simulink model "Example_VR_Simulation"  (Simulink 8.0)
settings: Solver=ode45  StartTime=0.0  StopTime=35  RelTol=1e-3
libraries: vrlib x6
settings Model: Creator=ajn5049  LastModifiedBy=ajn5049

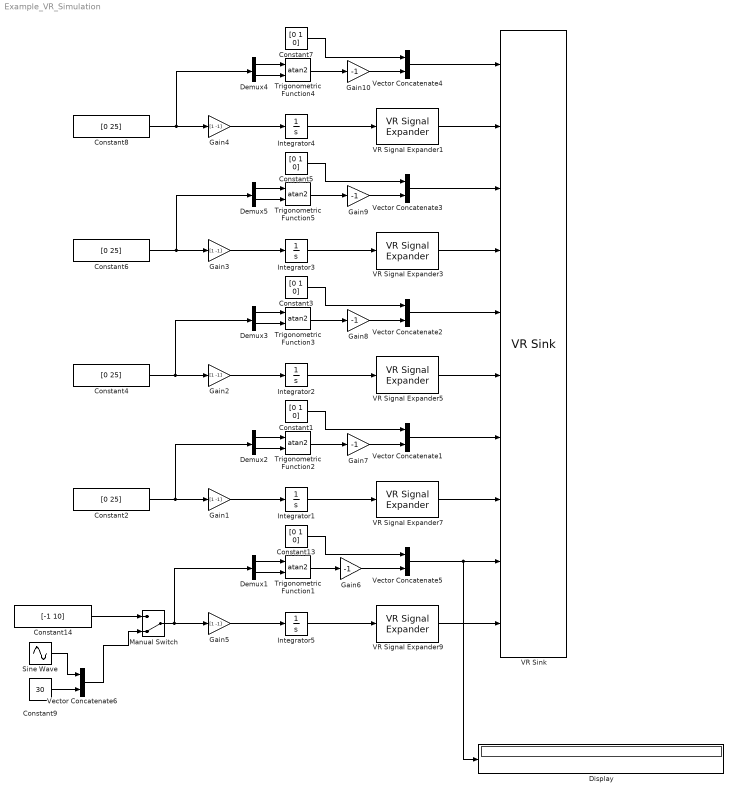
== system Example_VR_Simulation ==
  Constant{1,3,5,7,13} (5 alike) : Constant  Value=[0 1 0]
  Constant14 : Constant  Value=[-1 10]
  Constant{2,4,6,8} (4 alike) : Constant  Value=[0 25]
  Constant9 : Constant  Value=30
  Demux{1..5} (5 alike) : Demux  Outputs=2
  Display : Display
  Gain{1..5} (5 alike) : Gain  Gain=[1 -1]
  Gain{6..10} (5 alike) : Gain  Gain=-1
  Integrator{1..4} (4 alike) : Integrator  InitialCondition=[0, 0]
  Integrator5 : Integrator  InitialCondition=[-3.66/2, 0]
  Manual Switch : ManualSwitch  CurrentSetting=0
  Sine Wave : Sin  Amplitude=2  Phase=pi/2  SampleTime=0
  Trigonometric Function{1..5} (5 alike) : Trigonometry  Operator=atan2
  VR Signal Expander{1,3,5,7,9} (5 alike) : vrlib/VR Signal Expander  outwidth=3  outidx=[1 3]
  VR Sink : vrlib/VR Sink  InstantiateOnLoad=on  SampleTime=0.1  ViewEnable=on  RemoteChange=off  RemoteView=off  FieldsWritten=Lotus.rotation.4.1.1.double#Lotus.translation.3.1.1.double#Alfa_Romeo.rotation.4.1.1.double#Alfa_Romeo.translation.3.1.1.double#Logging_Truck.rotation.4.1.1.double#Logging_Truck.translation.3.1.1.double#Mustang.rotation.4.1.1.double#Mustang.translation.3.1.1.double#Octavia.rotation.4.1.1.double#Octavia.translation.3.1.1.double  WorldFileName=C:\Other\Virtual Worlds\VR_Simulation.wrl  WorldDescription=Simple Highway Model  AutoView=on  VideoDimensions=[200 320]*2  AllowVariableSize=off  FigureProperties="{'Position', 'Name', 'Viewpoint', 'CameraBound', 'CameraDirection', 'CameraPosition', 'CameraUpVector', 'ZoomFactor', 'Antialiasing', 'Headlight', 'Lighting', 'NavPanel', 'StatusBar', 'ToolBar', 'Textures', 'Transparency', 'Triad', 'Wireframe', 'NavZones', 'NavMode', 'NavSpeed', 'CaptureFileFormat', 'CaptureFileName', 'Record2DCompressMethod', 'Record2DCompressQuality', 'Record2D', 'Record2DFileName', 'Record2DFPS'; [5.0000000000000000e+00   9.2000000000000000e+01   5.7600000000000000e+02   3.8000000000000000e+02], 'Simple Highway Model', 'Car1 - View from Behind - Rot', 'on', [0.0000000000000000e+00   0.0000000000000000e+00  -1.0000000000000000e+00], [0.0000000000000000e+00   0.0000000000000000e+00   0.0000000000000000e+00], [0.0000000000000000e+00   1.0000000000000000e+00   0.0000000000000000e+00], [1.0000000000000000e+00], 'on', 'on', 'on', 'halfbar', 'on', 'on', 'on', 'on', 'none', 'off', 'off', 'walk', 'normal', 'tif', '%f_anim_%n.tif', 'auto', [7.5000000000000000e+01], 'off', '%f_anim_%n.avi', [1.5000000000000000e+01]; [5.8600000000000000e+02   6.0000000000000000e+01   6.4000000000000000e+02   4.0000000000000000e+02], 'Simple Highway Model', 'Car1 - View from Above Ahead - Rot', 'on', [0.0000000000000000e+00   0.0000000000000000e+00  -1.0000000000000000e+00], [0.0000000000000000e+00   0.0000000000000000e+00   0.0000000000000000e+00], [0.0000000000000000e+00   1.0000000000000000e+00   0.0000000000000000e+00], [1.0000000000000000e+00], 'on', 'on', 'on', 'none', 'off', 'off', 'on', 'on', 'none', 'off', 'off', 'walk', 'normal', 'tif', '%f_anim_%n.tif', 'auto', [7.5000000000000000e+01], 'off', '***video***', [1.5000000000000000e+01]}"
  Vector Concatenate{1..6} (6 alike) : Concatenate
  wires:
  Trigonometric Function1/1 -> Gain6/1
  Constant13/1 -> Vector Concatenate5/1
  Integrator5/1 -> VR Signal Expander9/1
  Gain5/1 -> Integrator5/1
  Vector Concatenate4/1 -> VR Sink/1
  Vector Concatenate1/1 -> VR Sink/7
  VR Signal Expander5/1 -> VR Sink/6
  VR Signal Expander7/1 -> VR Sink/8
  Vector Concatenate5/1 -> Display/1, VR Sink/9
  Vector Concatenate2/1 -> VR Sink/5
  VR Signal Expander3/1 -> VR Sink/4
  VR Signal Expander9/1 -> VR Sink/10
  Vector Concatenate3/1 -> VR Sink/3
  VR Signal Expander1/1 -> VR Sink/2
  Trigonometric Function2/1 -> Gain7/1
  Constant1/1 -> Vector Concatenate1/1
  Integrator1/1 -> VR Signal Expander7/1
  Gain1/1 -> Integrator1/1
  Trigonometric Function3/1 -> Gain8/1
  Constant3/1 -> Vector Concatenate2/1
  Integrator2/1 -> VR Signal Expander5/1
  Gain2/1 -> Integrator2/1
  Constant6/1 -> Demux5/1, Gain3/1
  Integrator3/1 -> VR Signal Expander3/1
  Gain3/1 -> Integrator3/1
  Trigonometric Function4/1 -> Gain10/1
  Constant7/1 -> Vector Concatenate4/1
  Constant8/1 -> Demux4/1, Gain4/1
  Integrator4/1 -> VR Signal Expander1/1
  Gain4/1 -> Integrator4/1
  Demux4/1 -> Trigonometric Function4/1
  Demux4/2 -> Trigonometric Function4/2
  Vector Concatenate6/1 -> Manual Switch/2
  Demux1/1 -> Trigonometric Function1/1
  Demux1/2 -> Trigonometric Function1/2
  Constant2/1 -> Demux2/1, Gain1/1
  Demux2/1 -> Trigonometric Function2/1
  Demux2/2 -> Trigonometric Function2/2
  Constant4/1 -> Demux3/1, Gain2/1
  Demux3/1 -> Trigonometric Function3/1
  Demux3/2 -> Trigonometric Function3/2
  Trigonometric Function5/1 -> Gain9/1
  Demux5/1 -> Trigonometric Function5/1
  Demux5/2 -> Trigonometric Function5/2
  Constant5/1 -> Vector Concatenate3/1
  Gain6/1 -> Vector Concatenate5/2
  Gain7/1 -> Vector Concatenate1/2
  Gain8/1 -> Vector Concatenate2/2
  Gain9/1 -> Vector Concatenate3/2
  Gain10/1 -> Vector Concatenate4/2
  Manual Switch/1 -> Demux1/1, Gain5/1
  Constant14/1 -> Manual Switch/1
  Constant9/1 -> Vector Concatenate6/2
  Sine Wave/1 -> Vector Concatenate6/1
